simulink model "FixedPointControll"  (R2020b)
settings: Solver=VariableStepAuto  StartTime=0.0  StopTime=300  RelTol=1e-3
values from neighbouring files (symbols this model uses):
  K = acker(A,B,poles)    [double_tank_init.m]
  V = -1/(C*inv(A-B*K)*B)    [double_tank_init.m]
undefined symbols (not defined in the file or in its folder): National_Instruments, PCIe
libraries: sldrtlib x3
settings Model: Creator=EAL  LastModifiedBy=EAL

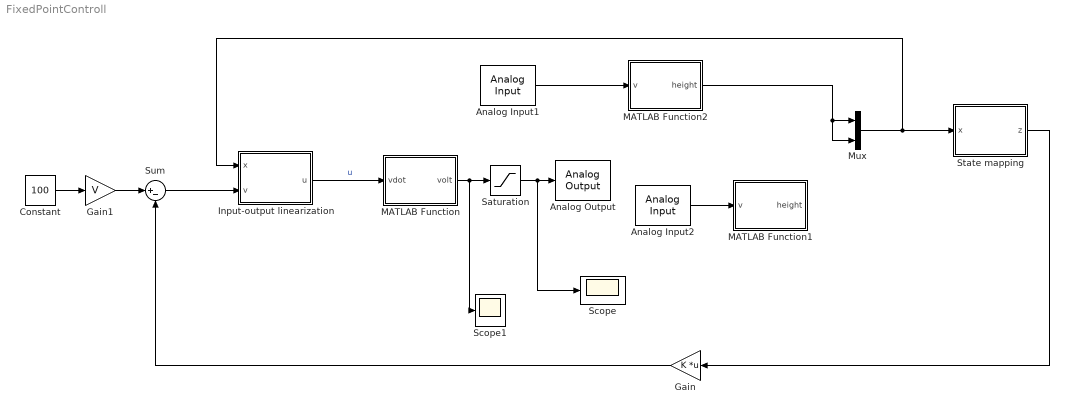
== system FixedPointControll ==
  Analog Input1 : sldrtlib/Analog Input  SampleTime=0.1  MaxMissedTicks=10  ShowMissedTicks=off  YieldWhenWaiting=off  DrvName=National_Instruments/PCIe-6321  DrvAddress=4294967295  DrvOptions=[0 0 0 0 0 0 0]  Channels=1  RangeMode=1  VoltRange=1  DataType=1
      settings: AttributesFormatString=National Instruments\nPCIe-6321 [auto]
  Analog Input2 : sldrtlib/Analog Input  SampleTime=0.1  MaxMissedTicks=10  ShowMissedTicks=off  YieldWhenWaiting=off  DrvName=National_Instruments/PCIe-6321  DrvAddress=4294967295  DrvOptions=[0 0 0 0 0 0 0]  Channels=1  RangeMode=1  VoltRange=1  DataType=1
      settings: AttributesFormatString=National Instruments\nPCIe-6321 [auto]
  Analog Output : sldrtlib/Analog Output  SampleTime=0.1  MaxMissedTicks=10  ShowMissedTicks=off  YieldWhenWaiting=off  DrvName=National_Instruments/PCIe-6321  DrvAddress=4294967295  DrvOptions=[0 0 0 0 0 0 0]  Channels=1  RangeMode=1  VoltRange=1  InitialValue=0  FinalValue=0
      settings: AttributesFormatString=National Instruments\nPCIe-6321 [auto]
  Constant : Constant  Value=100
  Gain : Gain  Gain=K  Multiplication=Matrix(K*u)
  Gain1 : Gain  Gain=V
  Input-output linearization : MATLAB Function  TreatAsAtomicUnit=on
  MATLAB Function : MATLAB Function  TreatAsAtomicUnit=on
  MATLAB Function1 : MATLAB Function  TreatAsAtomicUnit=on
  MATLAB Function2 : MATLAB Function  TreatAsAtomicUnit=on
  Mux : Mux  Inputs=2
  Saturation : Saturate  UpperLimit=10  LowerLimit=0
  Scope : Scope
  Scope1 : Scope
  State mapping : MATLAB Function  TreatAsAtomicUnit=on
  Sum : Sum  Inputs=|+-
  wires:
  Analog Input2/1 -> MATLAB Function1/1(v)
  Mux/1 -> Input-output linearization/1(x), State mapping/1(x)
  State mapping/1(z) -> Gain/1
  Gain/1 -> Sum/2
  Sum/1 -> Input-output linearization/2(v)
  Input-output linearization/1(u) -> MATLAB Function/1(vdot)  "u"
  MATLAB Function/1(volt) -> Scope1/1, Saturation/1
  Saturation/1 -> Scope/1, Analog Output/1
  Constant/1 -> Gain1/1
  Gain1/1 -> Sum/1
  Analog Input1/1 -> MATLAB Function2/1(v)
  MATLAB Function2/1(height) -> Mux/2, Mux/1

== matlab function FixedPointControll/State mapping ==
  data: x input; z output; p parameter
function z = fcn(x,p)
%#codegen
z = 0*x; % assignment before subscripting
z(1) = x(2);
z(2) = p.a*sqrt(x(1))-p.a*sqrt(x(2));

== matlab function FixedPointControll/Input-output linearization ==
  data: x input; v input; u output; p parameter
function u = fcn(x,v,p)
u = 0;
u = (1/16.666)*p.rho*p.At*sqrt(x(1))*(2*v/p.a+...
    p.a*sqrt(x(1))/sqrt(x(2)));

== matlab function FixedPointControll/MATLAB Function1 ==
  data: v input; height output
function height = fcn(v)

height = 115.3624*v-237.3624

== matlab function FixedPointControll/MATLAB Function ==
  data: vdot input; volt output
function volt = fcn(vdot)

volt = (1/100)*((-500/60)+16.666*vdot);

== matlab function FixedPointControll/MATLAB Function2 ==
  data: v input; height output
function height = fcn(v)

height = 115.3624*v-237.3624
